simulink model "butterfly"  (R2020a)
settings: Solver=VariableStepAuto  StartTime=0.0  StopTime=10.0  RelTol=1e-3
settings Model: Creator=g-oft  LastModifiedBy=g-oft

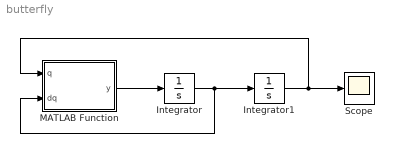
== system butterfly ==
  Integrator : Integrator  InitialCondition=[0;1.2]
  Integrator1 : Integrator  InitialCondition=[0;0]
  MATLAB Function : MATLAB Function  TreatAsAtomicUnit=on
  Scope : Scope
  wires:
  MATLAB Function/1(y) -> Integrator/1
  Integrator/1 -> MATLAB Function/2(dq), Integrator1/1
  Integrator1/1 -> MATLAB Function/1(q), Scope/1

== matlab function butterfly/MATLAB Function ==
  data: q input; y output; dq input
function y = fcn(q,dq)
    f = @(x,y) diff([x(2)+x(1)^2;y(1)^4],x);
y = f(q,dq);
